simulink library "myLibrary"  (R2023b)
settings: Solver=VariableStepAuto  StartTime=0.0  StopTime=10.0  RelTol=1e-3
undefined symbols (not defined in the file): Cac_n1, ctrl1, Da, delta_slk, Discrete, dtha, ee_sli_rtmsupport, FA, gcbh, Ha, Ini, init_DCline, init_IPC, init_line, init_load, init_SG, init_shunt, init_TH, init_trafo, init_user, init_VSC, initMachineBlocks, Ka, Lf, Llkd_pu, Llkq1_pu, magnitude, NET, P, plots_step, q0, Rac_n1, Radd, Rkd_pu, Rkq1_pu, Rload_add, sim_config, sps_rtmsupport, spsSteamTurbineModel, T_DC_NET, T_global, T_IPC, T_load, T_NET, T_SG, T_shunt, T_STATCOM, T_TH, T_trafo, T_user, T_VSC, Ts, tstep, Udiff_a, V1
libraries: spsSeriesRLCBranchLib x120, eeGeneralControl x83, $bdroot x78, spsCurrentMeasurementLib x53, spsParallelRLCBranchLib x39, spsVoltageMeasurementLib x37, spsControlledVoltageSourceLib x30, simulink x29, spsFirstOrderFilterLib x18, spsMeasurementModel x13, spsThreePhaseVIMeasurementLib x5, dspsigops x4
(part 16 of 16)

== system myLibrary/SG_step/Governor-Turbine/Steam Turbine and Governor/Model/4 mass shaft/3 masses/Mass4 ==
  note: implements discretized state-space model of mass dynamic equations using trapezoidal method
      |
      | x(k)= Ad*x(k-1) + Bd*(u(k)+u(k-1))
  note: In order to avoid an algebraic loop
      | the deltat_n(k-1) value is sent to output 1
      | instead of  deltat_n(k).
      | The delay is then compensated by a
      | linear extrapolatiom (Prediction bloc)
  note: Initialization of this delay is not required
      | because x(k) is initialized by IC switch block
  Ts_n+1 : Inport
  Tt_n : Inport  Port=2
  deltat_n-1 : Inport  Port=3
  Ad*x(k-1) : Gain  Gain=Ad  Multiplication=Matrix(K*u)  SaturateOnIntegerOverflow=on  SampleTime=Ts  OutDataTypeStr=Inherit: Same as input  ParamDataTypeStr=Inherit: Same as input
  Bd*(u(k)+ u(k-1)) : Gain  Gain=Bd  Multiplication=Matrix(K*u)  SaturateOnIntegerOverflow=on  SampleTime=Ts  OutDataTypeStr=Inherit: Same as input  ParamDataTypeStr=Inherit: Same as input
  Delay_u : UnitDelay  SampleTime=Ts  HasFrameUpgradeWarning=on
  Delay_x : UnitDelay  InitialCondition=[0 dth0]  SampleTime=Ts  HasFrameUpgradeWarning=on
  Demux : Demux  Outputs=2
  Demux1 : Demux  Outputs=2
  Digital Clock : DigitalClock  SampleTime=Ts
  Gain11 : Gain  Gain=K  SaturateOnIntegerOverflow=on  OutDataTypeStr=Inherit: Same as input  ParamDataTypeStr=Inherit: Same as input
  IC : Switch  Threshold=Ts  SaturateOnIntegerOverflow=off  InputSameDT=off
  Mux : Mux  Inputs=2
  Prediction : Subsystem
  Sum1 : Sum  Inputs=+-  InputSameDT=on  SaturateOnIntegerOverflow=on  OutDataTypeStr=Inherit: Same as first input
  Sum3 : Sum  InputSameDT=on  SaturateOnIntegerOverflow=on  OutDataTypeStr=Inherit: Same as first input
  Sum9 : Sum  InputSameDT=on  SaturateOnIntegerOverflow=on  OutDataTypeStr=Inherit: Same as first input
  Terminator : Terminator
  sum : Sum  SaturateOnIntegerOverflow=on
  deltat_n : Outport  InitialOutput=0
  "Ts_n " : Outport  Port=2  InitialOutput=0
  dw : Outport  Port=3  InitialOutput=0
  wires:
  Prediction/1(O) -> deltat_n/1
  Demux1/1 -> Terminator/1
  Demux1/2 -> Prediction/1(I)
  Demux/2 -> Sum1/1  "x2(k)"
  Demux/1 -> dw/1  "x1(k)"
  IC/1 -> Demux/1, Delay_x/1
  Sum3/1 -> IC/1  "x(k)"
  Digital Clock/1 -> IC/2
  Delay_x/1 -> Ad*x(k-1)/1, Demux1/1, IC/3  "x(k-1)"
  Ad*x(k-1)/1 -> Sum3/1
  Bd*(u(k)+ u(k-1))/1 -> Sum3/2
  sum/1 -> Bd*(u(k)+ u(k-1))/1  "u(k) + u(k-1)"
  Delay_u/1 -> sum/2
  Tt_n/1 -> Sum9/2
  Ts_n+1/1 -> Sum9/1
  Sum9/1 -> Mux/1  "u1 (k)"
  deltat_n-1/1 -> Sum1/2, Mux/2  "u2(k)"
  Mux/1 -> sum/1, Delay_u/1  "u(k)"
  Sum1/1 -> Gain11/1
  Gain11/1 -> "Ts_n "/1

== system myLibrary/SG_step/Governor-Turbine/Steam Turbine and Governor/Model/4 mass shaft/4 masses/Mass2 ==
  note: Initialization of this delay is not required
      | because x(k) is initialized by IC switch block
  note: In order to avoid an algebraic loop
      | the deltat_n(k-1) value is sent to output 1
      | instead of  deltat_n(k).
      | The delay is then compensated by a
      | linear extrapolatiom (Prediction bloc)
  note: implements discretized state-space model of mass dynamic equations using trapezoidal method
      |
      | x(k)= Ad*x(k-1) + Bd*(u(k)+u(k-1))
  Ts_n+1 : Inport
  Tt_n : Inport  Port=2
  deltat_n-1 : Inport  Port=3
  Ad*x(k-1) : Gain  Gain=Ad  Multiplication=Matrix(K*u)  SaturateOnIntegerOverflow=on  SampleTime=Ts  OutDataTypeStr=Inherit: Same as input  ParamDataTypeStr=Inherit: Same as input
  Bd*(u(k)+ u(k-1)) : Gain  Gain=Bd  Multiplication=Matrix(K*u)  SaturateOnIntegerOverflow=on  SampleTime=Ts  OutDataTypeStr=Inherit: Same as input  ParamDataTypeStr=Inherit: Same as input
  Delay_u : UnitDelay  SampleTime=Ts  HasFrameUpgradeWarning=on
  Delay_x : UnitDelay  InitialCondition=[0 initSG.delta2]  SampleTime=Ts  HasFrameUpgradeWarning=on
  Demux : Demux  Outputs=2
  Demux1 : Demux  Outputs=2
  Digital Clock : DigitalClock  SampleTime=Ts
  Gain11 : Gain  Gain=K  SaturateOnIntegerOverflow=on  OutDataTypeStr=Inherit: Same as input  ParamDataTypeStr=Inherit: Same as input
  IC : Switch  Threshold=Ts  SaturateOnIntegerOverflow=off  InputSameDT=off
  Mux : Mux  Inputs=2
  Prediction : Subsystem
  Sum1 : Sum  Inputs=+-  InputSameDT=on  SaturateOnIntegerOverflow=on  OutDataTypeStr=Inherit: Same as first input
  Sum3 : Sum  InputSameDT=on  SaturateOnIntegerOverflow=on  OutDataTypeStr=Inherit: Same as first input
  Sum9 : Sum  InputSameDT=on  SaturateOnIntegerOverflow=on  OutDataTypeStr=Inherit: Same as first input
  Terminator : Terminator
  sum : Sum  SaturateOnIntegerOverflow=on
  deltat_n : Outport  InitialOutput=0
  "Ts_n " : Outport  Port=2  InitialOutput=0
  dw : Outport  Port=3  InitialOutput=0
  wires:
  Gain11/1 -> "Ts_n "/1
  Sum1/1 -> Gain11/1
  Mux/1 -> Delay_u/1, sum/1  "u(k)"
  deltat_n-1/1 -> Mux/2, Sum1/2  "u2(k)"
  Sum9/1 -> Mux/1  "u1 (k)"
  Ts_n+1/1 -> Sum9/1
  Tt_n/1 -> Sum9/2
  Delay_u/1 -> sum/2
  sum/1 -> Bd*(u(k)+ u(k-1))/1  "u(k) + u(k-1)"
  Bd*(u(k)+ u(k-1))/1 -> Sum3/2
  Ad*x(k-1)/1 -> Sum3/1
  Delay_x/1 -> IC/3, Demux1/1, Ad*x(k-1)/1  "x(k-1)"
  Digital Clock/1 -> IC/2
  Sum3/1 -> IC/1  "x(k)"
  IC/1 -> Delay_x/1, Demux/1
  Demux/1 -> dw/1  "x1(k)"
  Demux/2 -> Sum1/1  "x2(k)"
  Demux1/2 -> Prediction/1(I)
  Demux1/1 -> Terminator/1
  Prediction/1(O) -> deltat_n/1

== system myLibrary/SG_step/Governor-Turbine/Steam Turbine and Governor/Model/4 mass shaft/4 masses/Mass3 ==
  note: implements discretized state-space model of mass dynamic equations using trapezoidal method
      |
      | x(k)= Ad*x(k-1) + Bd*(u(k)+u(k-1))
  note: In order to avoid an algebraic loop
      | the deltat_n(k-1) value is sent to output 1
      | instead of  deltat_n(k).
      | The delay is then compensated by a
      | linear extrapolatiom (Prediction bloc)
  note: Initialization of this delay is not required
      | because x(k) is initialized by IC switch block
  Ts_n+1 : Inport
  Tt_n : Inport  Port=2
  deltat_n-1 : Inport  Port=3
  Ad*x(k-1) : Gain  Gain=Ad  Multiplication=Matrix(K*u)  SaturateOnIntegerOverflow=on  SampleTime=Ts  OutDataTypeStr=Inherit: Same as input  ParamDataTypeStr=Inherit: Same as input
  Bd*(u(k)+ u(k-1)) : Gain  Gain=Bd  Multiplication=Matrix(K*u)  SaturateOnIntegerOverflow=on  SampleTime=Ts  OutDataTypeStr=Inherit: Same as input  ParamDataTypeStr=Inherit: Same as input
  Delay_u : UnitDelay  SampleTime=Ts  HasFrameUpgradeWarning=on
  Delay_x : UnitDelay  InitialCondition=[0 initSG.delta3]  SampleTime=Ts  HasFrameUpgradeWarning=on
  Demux : Demux  Outputs=2
  Demux1 : Demux  Outputs=2
  Digital Clock : DigitalClock  SampleTime=Ts
  Gain11 : Gain  Gain=K  SaturateOnIntegerOverflow=on  OutDataTypeStr=Inherit: Same as input  ParamDataTypeStr=Inherit: Same as input
  IC : Switch  Threshold=Ts  SaturateOnIntegerOverflow=off  InputSameDT=off
  Mux : Mux  Inputs=2
  Prediction : Subsystem
  Sum1 : Sum  Inputs=+-  InputSameDT=on  SaturateOnIntegerOverflow=on  OutDataTypeStr=Inherit: Same as first input
  Sum3 : Sum  InputSameDT=on  SaturateOnIntegerOverflow=on  OutDataTypeStr=Inherit: Same as first input
  Sum9 : Sum  InputSameDT=on  SaturateOnIntegerOverflow=on  OutDataTypeStr=Inherit: Same as first input
  Terminator : Terminator
  sum : Sum  SaturateOnIntegerOverflow=on
  deltat_n : Outport  InitialOutput=0
  "Ts_n " : Outport  Port=2  InitialOutput=0
  dw : Outport  Port=3  InitialOutput=0
  wires:
  Prediction/1(O) -> deltat_n/1
  Demux1/1 -> Terminator/1
  Demux1/2 -> Prediction/1(I)
  Demux/2 -> Sum1/1  "x2(k)"
  Demux/1 -> dw/1  "x1(k)"
  IC/1 -> Demux/1, Delay_x/1
  Sum3/1 -> IC/1  "x(k)"
  Digital Clock/1 -> IC/2
  Delay_x/1 -> Ad*x(k-1)/1, Demux1/1, IC/3  "x(k-1)"
  Ad*x(k-1)/1 -> Sum3/1
  Bd*(u(k)+ u(k-1))/1 -> Sum3/2
  sum/1 -> Bd*(u(k)+ u(k-1))/1  "u(k) + u(k-1)"
  Delay_u/1 -> sum/2
  Tt_n/1 -> Sum9/2
  Ts_n+1/1 -> Sum9/1
  Sum9/1 -> Mux/1  "u1 (k)"
  deltat_n-1/1 -> Sum1/2, Mux/2  "u2(k)"
  Mux/1 -> sum/1, Delay_u/1  "u(k)"
  Sum1/1 -> Gain11/1
  Gain11/1 -> "Ts_n "/1

== system myLibrary/SG_step/Governor-Turbine/Steam Turbine and Governor/Model/4 mass shaft/4 masses/Mass4 ==
  note: Initialization of this delay is not required
      | because x(k) is initialized by IC switch block
  note: In order to avoid an algebraic loop
      | the deltat_n(k-1) value is sent to output 1
      | instead of  deltat_n(k).
      | The delay is then compensated by a
      | linear extrapolatiom (Prediction bloc)
  note: implements discretized state-space model of mass dynamic equations using trapezoidal method
      |
      | x(k)= Ad*x(k-1) + Bd*(u(k)+u(k-1))
  Ts_n+1 : Inport
  Tt_n : Inport  Port=2
  deltat_n-1 : Inport  Port=3
  Ad*x(k-1) : Gain  Gain=Ad  Multiplication=Matrix(K*u)  SaturateOnIntegerOverflow=on  SampleTime=Ts  OutDataTypeStr=Inherit: Same as input  ParamDataTypeStr=Inherit: Same as input
  Bd*(u(k)+ u(k-1)) : Gain  Gain=Bd  Multiplication=Matrix(K*u)  SaturateOnIntegerOverflow=on  SampleTime=Ts  OutDataTypeStr=Inherit: Same as input  ParamDataTypeStr=Inherit: Same as input
  Delay_u : UnitDelay  SampleTime=Ts  HasFrameUpgradeWarning=on
  Delay_x : UnitDelay  InitialCondition=[0 initSG.delta4]  SampleTime=Ts  HasFrameUpgradeWarning=on
  Demux : Demux  Outputs=2
  Demux1 : Demux  Outputs=2
  Digital Clock : DigitalClock  SampleTime=Ts
  Gain11 : Gain  Gain=K  SaturateOnIntegerOverflow=on  OutDataTypeStr=Inherit: Same as input  ParamDataTypeStr=Inherit: Same as input
  IC : Switch  Threshold=Ts  SaturateOnIntegerOverflow=off  InputSameDT=off
  Mux : Mux  Inputs=2
  Prediction : Subsystem
  Sum1 : Sum  Inputs=+-  InputSameDT=on  SaturateOnIntegerOverflow=on  OutDataTypeStr=Inherit: Same as first input
  Sum3 : Sum  InputSameDT=on  SaturateOnIntegerOverflow=on  OutDataTypeStr=Inherit: Same as first input
  Sum9 : Sum  InputSameDT=on  SaturateOnIntegerOverflow=on  OutDataTypeStr=Inherit: Same as first input
  Terminator : Terminator
  sum : Sum  SaturateOnIntegerOverflow=on
  deltat_n : Outport  InitialOutput=0
  "Ts_n " : Outport  Port=2  InitialOutput=0
  dw : Outport  Port=3  InitialOutput=0
  wires:
  Gain11/1 -> "Ts_n "/1
  Sum1/1 -> Gain11/1
  Mux/1 -> Delay_u/1, sum/1  "u(k)"
  deltat_n-1/1 -> Mux/2, Sum1/2  "u2(k)"
  Sum9/1 -> Mux/1  "u1 (k)"
  Ts_n+1/1 -> Sum9/1
  Tt_n/1 -> Sum9/2
  Delay_u/1 -> sum/2
  sum/1 -> Bd*(u(k)+ u(k-1))/1  "u(k) + u(k-1)"
  Bd*(u(k)+ u(k-1))/1 -> Sum3/2
  Ad*x(k-1)/1 -> Sum3/1
  Delay_x/1 -> IC/3, Demux1/1, Ad*x(k-1)/1  "x(k-1)"
  Digital Clock/1 -> IC/2
  Sum3/1 -> IC/1  "x(k)"
  IC/1 -> Delay_x/1, Demux/1
  Demux/1 -> dw/1  "x1(k)"
  Demux/2 -> Sum1/1  "x2(k)"
  Demux1/2 -> Prediction/1(I)
  Demux1/1 -> Terminator/1
  Prediction/1(O) -> deltat_n/1

== system myLibrary/SG_step/Governor-Turbine/Steam Turbine and Governor/Model/4 mass shaft/4 masses/Mass5 ==
  note: implements discretized state-space model of mass dynamic equations using trapezoidal method
      |
      | x(k)= Ad*x(k-1) + Bd*(u(k)+u(k-1))
  note: In order to avoid an algebraic loop
      | the deltat_n(k-1) value is sent to output 1
      | instead of  deltat_n(k).
      | The delay is then compensated by a
      | linear extrapolatiom (Prediction bloc)
  note: Initialization of this delay is not required
      | because x(k) is initialized by IC switch block
  Ts_n+1 : Inport
  Tt_n : Inport  Port=2
  deltat_n-1 : Inport  Port=3
  Ad*x(k-1) : Gain  Gain=Ad  Multiplication=Matrix(K*u)  SaturateOnIntegerOverflow=on  SampleTime=Ts  OutDataTypeStr=Inherit: Same as input  ParamDataTypeStr=Inherit: Same as input
  Bd*(u(k)+ u(k-1)) : Gain  Gain=Bd  Multiplication=Matrix(K*u)  SaturateOnIntegerOverflow=on  SampleTime=Ts  OutDataTypeStr=Inherit: Same as input  ParamDataTypeStr=Inherit: Same as input
  Delay_u : UnitDelay  SampleTime=Ts  HasFrameUpgradeWarning=on
  Delay_x : UnitDelay  InitialCondition=[0 initSG.delta5]  SampleTime=Ts  HasFrameUpgradeWarning=on
  Demux : Demux  Outputs=2
  Demux1 : Demux  Outputs=2
  Digital Clock : DigitalClock  SampleTime=Ts
  Gain11 : Gain  Gain=K  SaturateOnIntegerOverflow=on  OutDataTypeStr=Inherit: Same as input  ParamDataTypeStr=Inherit: Same as input
  IC : Switch  Threshold=Ts  SaturateOnIntegerOverflow=off  InputSameDT=off
  Mux : Mux  Inputs=2
  Prediction : Subsystem
  Sum1 : Sum  Inputs=+-  InputSameDT=on  SaturateOnIntegerOverflow=on  OutDataTypeStr=Inherit: Same as first input
  Sum3 : Sum  InputSameDT=on  SaturateOnIntegerOverflow=on  OutDataTypeStr=Inherit: Same as first input
  Sum9 : Sum  InputSameDT=on  SaturateOnIntegerOverflow=on  OutDataTypeStr=Inherit: Same as first input
  Terminator : Terminator
  sum : Sum  SaturateOnIntegerOverflow=on
  deltat_n : Outport  InitialOutput=0
  "Ts_n " : Outport  Port=2  InitialOutput=0
  dw : Outport  Port=3  InitialOutput=0
  wires:
  Prediction/1(O) -> deltat_n/1
  Demux1/1 -> Terminator/1
  Demux1/2 -> Prediction/1(I)
  Demux/2 -> Sum1/1  "x2(k)"
  Demux/1 -> dw/1  "x1(k)"
  IC/1 -> Demux/1, Delay_x/1
  Sum3/1 -> IC/1  "x(k)"
  Digital Clock/1 -> IC/2
  Delay_x/1 -> Ad*x(k-1)/1, Demux1/1, IC/3  "x(k-1)"
  Ad*x(k-1)/1 -> Sum3/1
  Bd*(u(k)+ u(k-1))/1 -> Sum3/2
  sum/1 -> Bd*(u(k)+ u(k-1))/1  "u(k) + u(k-1)"
  Delay_u/1 -> sum/2
  Tt_n/1 -> Sum9/2
  Ts_n+1/1 -> Sum9/1
  Sum9/1 -> Mux/1  "u1 (k)"
  deltat_n-1/1 -> Sum1/2, Mux/2  "u2(k)"
  Mux/1 -> sum/1, Delay_u/1  "u(k)"
  Sum1/1 -> Gain11/1
  Gain11/1 -> "Ts_n "/1

== system myLibrary/SG_step/Governor-Turbine/Steam Turbine and Governor/Model/steam turbine MM/Stage 1/Stage1 ==
  In1 : Inport
  Enable : EnablePort
  Stage1 : spsFirstOrderFilterLib/First-Order Filter  FilterType=Lowpass  Tc=T1  Ts=Ts  Initialize=on  Vac_Init=[0, 0, 60]  Vdc_Init=f0  PlotResponse=off  FreqRange="[0,  200,  1]"
  Out1 : Outport  OutputWhenDisabled=reset  InitialOutput=0
  wires:
  In1/1 -> Stage1/1
  Stage1/1 -> Out1/1

== system myLibrary/SG_step/Governor-Turbine/Steam Turbine and Governor/Model/steam turbine MM/Stage 2 /Stage2 ==
  In1 : Inport
  Enable : EnablePort
  Stage2 : spsFirstOrderFilterLib/First-Order Filter  FilterType=Lowpass  Tc=T2  Ts=Ts  Initialize=on  Vac_Init=[0, 0, 60]  Vdc_Init=f0  PlotResponse=off  FreqRange="[0,  200,  1]"
  Out1 : Outport  OutputWhenDisabled=reset  InitialOutput=0
  wires:
  Stage2/1 -> Out1/1
  In1/1 -> Stage2/1

== system myLibrary/SG_step/Governor-Turbine/Steam Turbine and Governor/Model/steam turbine MM/Stage 3/Stage3 ==
  In1 : Inport
  Enable : EnablePort
  Stage3 : spsFirstOrderFilterLib/First-Order Filter  FilterType=Lowpass  Tc=T3  Ts=Ts  Initialize=on  Vac_Init=[0, 0, 60]  Vdc_Init=f0  PlotResponse=off  FreqRange="[0,  200,  1]"
  Out1 : Outport  OutputWhenDisabled=reset  InitialOutput=0
  wires:
  In1/1 -> Stage3/1
  Stage3/1 -> Out1/1

== system myLibrary/SG_step/Governor-Turbine/Steam Turbine and Governor/Model/steam turbine MM/Stage 4/Stage4 ==
  In1 : Inport
  Enable : EnablePort
  Stage4 : spsFirstOrderFilterLib/First-Order Filter  FilterType=Lowpass  Tc=T4  Ts=Ts  Initialize=on  Vac_Init=[0, 0, 60]  Vdc_Init=f0  PlotResponse=off  FreqRange="[0,  200,  1]"
  Out1 : Outport  OutputWhenDisabled=reset  InitialOutput=0
  wires:
  Stage4/1 -> Out1/1
  In1/1 -> Stage4/1

== system myLibrary/SG/Governor-Turbine/Steam Turbine and Governor/Model/4 mass shaft/1 mass/Mass2/Prediction ==
  I : Inport
  Gain1 : Gain  Gain=2  SaturateOnIntegerOverflow=on  OutDataTypeStr=Inherit: Same as input  ParamDataTypeStr=Inherit: Same as input
  Sum1 : Sum  Inputs=+-  InputSameDT=on  SaturateOnIntegerOverflow=on  OutDataTypeStr=Inherit: Same as first input
  Unit Delay3 : UnitDelay  InitialCondition=dth0  SampleTime=Ts  HasFrameUpgradeWarning=on
  O : Outport
  wires:
  Sum1/1 -> O/1
  Unit Delay3/1 -> Sum1/2
  Gain1/1 -> Sum1/1
  I/1 -> Unit Delay3/1, Gain1/1

== system myLibrary/SG/Governor-Turbine/Steam Turbine and Governor/Model/4 mass shaft/2 masses/Mass2/Prediction ==
  I : Inport
  Gain1 : Gain  Gain=2  SaturateOnIntegerOverflow=on  OutDataTypeStr=Inherit: Same as input  ParamDataTypeStr=Inherit: Same as input
  Sum1 : Sum  Inputs=+-  InputSameDT=on  SaturateOnIntegerOverflow=on  OutDataTypeStr=Inherit: Same as first input
  Unit Delay3 : UnitDelay  InitialCondition=dth0  SampleTime=Ts  HasFrameUpgradeWarning=on
  O : Outport
  wires:
  I/1 -> Gain1/1, Unit Delay3/1
  Gain1/1 -> Sum1/1
  Unit Delay3/1 -> Sum1/2
  Sum1/1 -> O/1

== system myLibrary/SG/Governor-Turbine/Steam Turbine and Governor/Model/4 mass shaft/2 masses/Mass3/Prediction ==
  I : Inport
  Gain1 : Gain  Gain=2  SaturateOnIntegerOverflow=on  OutDataTypeStr=Inherit: Same as input  ParamDataTypeStr=Inherit: Same as input
  Sum1 : Sum  Inputs=+-  InputSameDT=on  SaturateOnIntegerOverflow=on  OutDataTypeStr=Inherit: Same as first input
  Unit Delay3 : UnitDelay  InitialCondition=dth0  SampleTime=Ts  HasFrameUpgradeWarning=on
  O : Outport
  wires:
  Sum1/1 -> O/1
  Unit Delay3/1 -> Sum1/2
  Gain1/1 -> Sum1/1
  I/1 -> Unit Delay3/1, Gain1/1

== system myLibrary/SG/Governor-Turbine/Steam Turbine and Governor/Model/4 mass shaft/3 masses/Mass2/Prediction ==
  I : Inport
  Gain1 : Gain  Gain=2  SaturateOnIntegerOverflow=on  OutDataTypeStr=Inherit: Same as input  ParamDataTypeStr=Inherit: Same as input
  Sum1 : Sum  Inputs=+-  InputSameDT=on  SaturateOnIntegerOverflow=on  OutDataTypeStr=Inherit: Same as first input
  Unit Delay3 : UnitDelay  InitialCondition=dth0  SampleTime=Ts  HasFrameUpgradeWarning=on
  O : Outport
  wires:
  Sum1/1 -> O/1
  Unit Delay3/1 -> Sum1/2
  Gain1/1 -> Sum1/1
  I/1 -> Unit Delay3/1, Gain1/1

== system myLibrary/SG/Governor-Turbine/Steam Turbine and Governor/Model/4 mass shaft/3 masses/Mass3/Prediction ==
  I : Inport
  Gain1 : Gain  Gain=2  SaturateOnIntegerOverflow=on  OutDataTypeStr=Inherit: Same as input  ParamDataTypeStr=Inherit: Same as input
  Sum1 : Sum  Inputs=+-  InputSameDT=on  SaturateOnIntegerOverflow=on  OutDataTypeStr=Inherit: Same as first input
  Unit Delay3 : UnitDelay  InitialCondition=dth0  SampleTime=Ts  HasFrameUpgradeWarning=on
  O : Outport
  wires:
  I/1 -> Gain1/1, Unit Delay3/1
  Gain1/1 -> Sum1/1
  Unit Delay3/1 -> Sum1/2
  Sum1/1 -> O/1

== system myLibrary/SG/Governor-Turbine/Steam Turbine and Governor/Model/4 mass shaft/3 masses/Mass4/Prediction ==
  I : Inport
  Gain1 : Gain  Gain=2  SaturateOnIntegerOverflow=on  OutDataTypeStr=Inherit: Same as input  ParamDataTypeStr=Inherit: Same as input
  Sum1 : Sum  Inputs=+-  InputSameDT=on  SaturateOnIntegerOverflow=on  OutDataTypeStr=Inherit: Same as first input
  Unit Delay3 : UnitDelay  InitialCondition=dth0  SampleTime=Ts  HasFrameUpgradeWarning=on
  O : Outport
  wires:
  Sum1/1 -> O/1
  Unit Delay3/1 -> Sum1/2
  Gain1/1 -> Sum1/1
  I/1 -> Unit Delay3/1, Gain1/1

== system myLibrary/SG/Governor-Turbine/Steam Turbine and Governor/Model/4 mass shaft/4 masses/Mass2/Prediction ==
  I : Inport
  Gain1 : Gain  Gain=2  SaturateOnIntegerOverflow=on  OutDataTypeStr=Inherit: Same as input  ParamDataTypeStr=Inherit: Same as input
  Sum1 : Sum  Inputs=+-  InputSameDT=on  SaturateOnIntegerOverflow=on  OutDataTypeStr=Inherit: Same as first input
  Unit Delay3 : UnitDelay  InitialCondition=initSG.delta2  SampleTime=Ts  HasFrameUpgradeWarning=on
  O : Outport
  wires:
  I/1 -> Gain1/1, Unit Delay3/1
  Gain1/1 -> Sum1/1
  Unit Delay3/1 -> Sum1/2
  Sum1/1 -> O/1

== system myLibrary/SG/Governor-Turbine/Steam Turbine and Governor/Model/4 mass shaft/4 masses/Mass3/Prediction ==
  I : Inport
  Gain1 : Gain  Gain=2  SaturateOnIntegerOverflow=on  OutDataTypeStr=Inherit: Same as input  ParamDataTypeStr=Inherit: Same as input
  Sum1 : Sum  Inputs=+-  InputSameDT=on  SaturateOnIntegerOverflow=on  OutDataTypeStr=Inherit: Same as first input
  Unit Delay3 : UnitDelay  InitialCondition=initSG.delta3  SampleTime=Ts  HasFrameUpgradeWarning=on
  O : Outport
  wires:
  Sum1/1 -> O/1
  Unit Delay3/1 -> Sum1/2
  Gain1/1 -> Sum1/1
  I/1 -> Unit Delay3/1, Gain1/1

== system myLibrary/SG/Governor-Turbine/Steam Turbine and Governor/Model/4 mass shaft/4 masses/Mass4/Prediction ==
  I : Inport
  Gain1 : Gain  Gain=2  SaturateOnIntegerOverflow=on  OutDataTypeStr=Inherit: Same as input  ParamDataTypeStr=Inherit: Same as input
  Sum1 : Sum  Inputs=+-  InputSameDT=on  SaturateOnIntegerOverflow=on  OutDataTypeStr=Inherit: Same as first input
  Unit Delay3 : UnitDelay  InitialCondition=initSG.delta4  SampleTime=Ts  HasFrameUpgradeWarning=on
  O : Outport
  wires:
  I/1 -> Gain1/1, Unit Delay3/1
  Gain1/1 -> Sum1/1
  Unit Delay3/1 -> Sum1/2
  Sum1/1 -> O/1

== system myLibrary/SG/Governor-Turbine/Steam Turbine and Governor/Model/4 mass shaft/4 masses/Mass5/Prediction ==
  I : Inport
  Gain1 : Gain  Gain=2  SaturateOnIntegerOverflow=on  OutDataTypeStr=Inherit: Same as input  ParamDataTypeStr=Inherit: Same as input
  Sum1 : Sum  Inputs=+-  InputSameDT=on  SaturateOnIntegerOverflow=on  OutDataTypeStr=Inherit: Same as first input
  Unit Delay3 : UnitDelay  InitialCondition=initSG.delta5  SampleTime=Ts  HasFrameUpgradeWarning=on
  O : Outport
  wires:
  Sum1/1 -> O/1
  Unit Delay3/1 -> Sum1/2
  Gain1/1 -> Sum1/1
  I/1 -> Unit Delay3/1, Gain1/1

== system myLibrary/SG_step/Governor-Turbine/Steam Turbine and Governor/Model/4 mass shaft/1 mass/Mass2/Prediction ==
  I : Inport
  Gain1 : Gain  Gain=2  SaturateOnIntegerOverflow=on  OutDataTypeStr=Inherit: Same as input  ParamDataTypeStr=Inherit: Same as input
  Sum1 : Sum  Inputs=+-  InputSameDT=on  SaturateOnIntegerOverflow=on  OutDataTypeStr=Inherit: Same as first input
  Unit Delay3 : UnitDelay  InitialCondition=dth0  SampleTime=Ts  HasFrameUpgradeWarning=on
  O : Outport
  wires:
  Sum1/1 -> O/1
  Unit Delay3/1 -> Sum1/2
  Gain1/1 -> Sum1/1
  I/1 -> Unit Delay3/1, Gain1/1

== system myLibrary/SG_step/Governor-Turbine/Steam Turbine and Governor/Model/4 mass shaft/2 masses/Mass2/Prediction ==
  I : Inport
  Gain1 : Gain  Gain=2  SaturateOnIntegerOverflow=on  OutDataTypeStr=Inherit: Same as input  ParamDataTypeStr=Inherit: Same as input
  Sum1 : Sum  Inputs=+-  InputSameDT=on  SaturateOnIntegerOverflow=on  OutDataTypeStr=Inherit: Same as first input
  Unit Delay3 : UnitDelay  InitialCondition=dth0  SampleTime=Ts  HasFrameUpgradeWarning=on
  O : Outport
  wires:
  I/1 -> Gain1/1, Unit Delay3/1
  Gain1/1 -> Sum1/1
  Unit Delay3/1 -> Sum1/2
  Sum1/1 -> O/1

== system myLibrary/SG_step/Governor-Turbine/Steam Turbine and Governor/Model/4 mass shaft/2 masses/Mass3/Prediction ==
  I : Inport
  Gain1 : Gain  Gain=2  SaturateOnIntegerOverflow=on  OutDataTypeStr=Inherit: Same as input  ParamDataTypeStr=Inherit: Same as input
  Sum1 : Sum  Inputs=+-  InputSameDT=on  SaturateOnIntegerOverflow=on  OutDataTypeStr=Inherit: Same as first input
  Unit Delay3 : UnitDelay  InitialCondition=dth0  SampleTime=Ts  HasFrameUpgradeWarning=on
  O : Outport
  wires:
  Sum1/1 -> O/1
  Unit Delay3/1 -> Sum1/2
  Gain1/1 -> Sum1/1
  I/1 -> Unit Delay3/1, Gain1/1

== system myLibrary/SG_step/Governor-Turbine/Steam Turbine and Governor/Model/4 mass shaft/3 masses/Mass2/Prediction ==
  I : Inport
  Gain1 : Gain  Gain=2  SaturateOnIntegerOverflow=on  OutDataTypeStr=Inherit: Same as input  ParamDataTypeStr=Inherit: Same as input
  Sum1 : Sum  Inputs=+-  InputSameDT=on  SaturateOnIntegerOverflow=on  OutDataTypeStr=Inherit: Same as first input
  Unit Delay3 : UnitDelay  InitialCondition=dth0  SampleTime=Ts  HasFrameUpgradeWarning=on
  O : Outport
  wires:
  Sum1/1 -> O/1
  Unit Delay3/1 -> Sum1/2
  Gain1/1 -> Sum1/1
  I/1 -> Unit Delay3/1, Gain1/1

== system myLibrary/SG_step/Governor-Turbine/Steam Turbine and Governor/Model/4 mass shaft/3 masses/Mass3/Prediction ==
  I : Inport
  Gain1 : Gain  Gain=2  SaturateOnIntegerOverflow=on  OutDataTypeStr=Inherit: Same as input  ParamDataTypeStr=Inherit: Same as input
  Sum1 : Sum  Inputs=+-  InputSameDT=on  SaturateOnIntegerOverflow=on  OutDataTypeStr=Inherit: Same as first input
  Unit Delay3 : UnitDelay  InitialCondition=dth0  SampleTime=Ts  HasFrameUpgradeWarning=on
  O : Outport
  wires:
  I/1 -> Gain1/1, Unit Delay3/1
  Gain1/1 -> Sum1/1
  Unit Delay3/1 -> Sum1/2
  Sum1/1 -> O/1

== system myLibrary/SG_step/Governor-Turbine/Steam Turbine and Governor/Model/4 mass shaft/3 masses/Mass4/Prediction ==
  I : Inport
  Gain1 : Gain  Gain=2  SaturateOnIntegerOverflow=on  OutDataTypeStr=Inherit: Same as input  ParamDataTypeStr=Inherit: Same as input
  Sum1 : Sum  Inputs=+-  InputSameDT=on  SaturateOnIntegerOverflow=on  OutDataTypeStr=Inherit: Same as first input
  Unit Delay3 : UnitDelay  InitialCondition=dth0  SampleTime=Ts  HasFrameUpgradeWarning=on
  O : Outport
  wires:
  Sum1/1 -> O/1
  Unit Delay3/1 -> Sum1/2
  Gain1/1 -> Sum1/1
  I/1 -> Unit Delay3/1, Gain1/1

== system myLibrary/SG_step/Governor-Turbine/Steam Turbine and Governor/Model/4 mass shaft/4 masses/Mass2/Prediction ==
  I : Inport
  Gain1 : Gain  Gain=2  SaturateOnIntegerOverflow=on  OutDataTypeStr=Inherit: Same as input  ParamDataTypeStr=Inherit: Same as input
  Sum1 : Sum  Inputs=+-  InputSameDT=on  SaturateOnIntegerOverflow=on  OutDataTypeStr=Inherit: Same as first input
  Unit Delay3 : UnitDelay  InitialCondition=initSG.delta2  SampleTime=Ts  HasFrameUpgradeWarning=on
  O : Outport
  wires:
  I/1 -> Gain1/1, Unit Delay3/1
  Gain1/1 -> Sum1/1
  Unit Delay3/1 -> Sum1/2
  Sum1/1 -> O/1

== system myLibrary/SG_step/Governor-Turbine/Steam Turbine and Governor/Model/4 mass shaft/4 masses/Mass3/Prediction ==
  I : Inport
  Gain1 : Gain  Gain=2  SaturateOnIntegerOverflow=on  OutDataTypeStr=Inherit: Same as input  ParamDataTypeStr=Inherit: Same as input
  Sum1 : Sum  Inputs=+-  InputSameDT=on  SaturateOnIntegerOverflow=on  OutDataTypeStr=Inherit: Same as first input
  Unit Delay3 : UnitDelay  InitialCondition=initSG.delta3  SampleTime=Ts  HasFrameUpgradeWarning=on
  O : Outport
  wires:
  Sum1/1 -> O/1
  Unit Delay3/1 -> Sum1/2
  Gain1/1 -> Sum1/1
  I/1 -> Unit Delay3/1, Gain1/1

== system myLibrary/SG_step/Governor-Turbine/Steam Turbine and Governor/Model/4 mass shaft/4 masses/Mass4/Prediction ==
  I : Inport
  Gain1 : Gain  Gain=2  SaturateOnIntegerOverflow=on  OutDataTypeStr=Inherit: Same as input  ParamDataTypeStr=Inherit: Same as input
  Sum1 : Sum  Inputs=+-  InputSameDT=on  SaturateOnIntegerOverflow=on  OutDataTypeStr=Inherit: Same as first input
  Unit Delay3 : UnitDelay  InitialCondition=initSG.delta4  SampleTime=Ts  HasFrameUpgradeWarning=on
  O : Outport
  wires:
  I/1 -> Gain1/1, Unit Delay3/1
  Gain1/1 -> Sum1/1
  Unit Delay3/1 -> Sum1/2
  Sum1/1 -> O/1

== system myLibrary/SG_step/Governor-Turbine/Steam Turbine and Governor/Model/4 mass shaft/4 masses/Mass5/Prediction ==
  I : Inport
  Gain1 : Gain  Gain=2  SaturateOnIntegerOverflow=on  OutDataTypeStr=Inherit: Same as input  ParamDataTypeStr=Inherit: Same as input
  Sum1 : Sum  Inputs=+-  InputSameDT=on  SaturateOnIntegerOverflow=on  OutDataTypeStr=Inherit: Same as first input
  Unit Delay3 : UnitDelay  InitialCondition=initSG.delta5  SampleTime=Ts  HasFrameUpgradeWarning=on
  O : Outport
  wires:
  Sum1/1 -> O/1
  Unit Delay3/1 -> Sum1/2
  Gain1/1 -> Sum1/1
  I/1 -> Unit Delay3/1, Gain1/1

== matlab function myLibrary/SG/Exciter/Exciter ST4B/Fex/fex ==
  data: I_N input; F_EX output
function F_EX = fex(I_N)
% AVRFEX Rectifier regulation characteristic based on: IEEE Recommended
% Practice for Excitation System Models for Power System Stability Studies,
% IEEE Std 421.5-2006,Annex D, Rectifier Regulation

F_EX = ee.control.sm.fex(I_N);

end

== matlab function myLibrary/SG_step/Exciter/Exciter ST4B/Fex/fex ==
  data: I_N input; F_EX output
function F_EX = fex(I_N)
% AVRFEX Rectifier regulation characteristic based on: IEEE Recommended
% Practice for Excitation System Models for Power System Stability Studies,
% IEEE Std 421.5-2006,Annex D, Rectifier Regulation

F_EX = ee.control.sm.fex(I_N);

end
